simulink library "lib_Fin_Deflections"  (R2018b)
settings: Solver=VariableStepAuto  StartTime=0.0  StopTime=10.0  RelTol=1e-3
undefined symbols (not defined in the file or in its folder): FCC_PIX_Data, HIL_Data
settings Model: Creator=m.hiepp  LastModifiedBy=m.hiepp

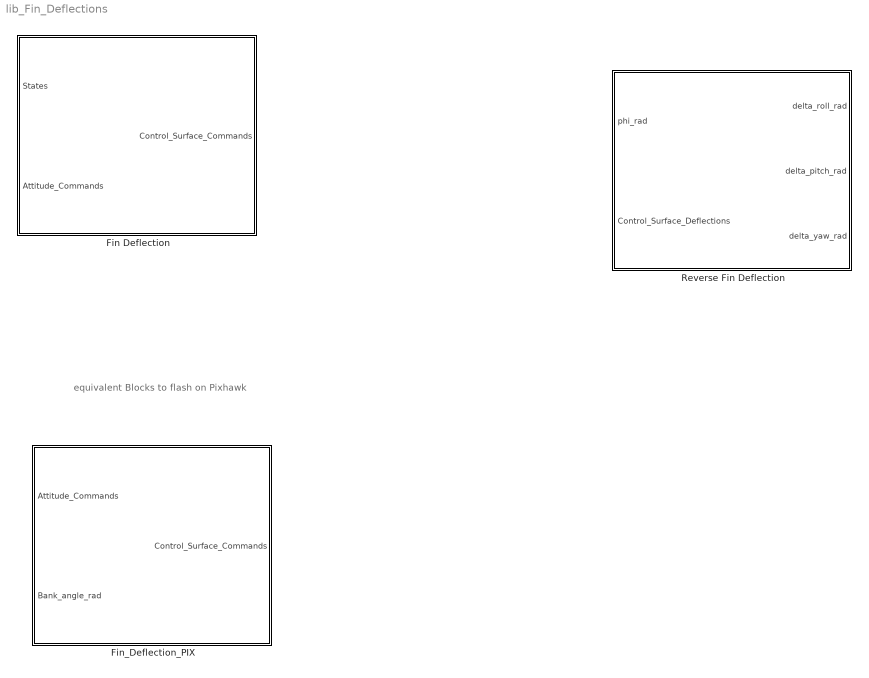
== system lib_Fin_Deflections ==
  note: equivalent Blocks to flash on Pixhawk
  Fin Deflection : Subsystem  mask{Control_Surfaces=HIL_Data.Control_Surfaces}
  Fin_Deflection_PIX : Subsystem
  Reverse Fin Deflection : Subsystem  mask{Control_Surfaces=HIL_Data.Control_Surfaces}

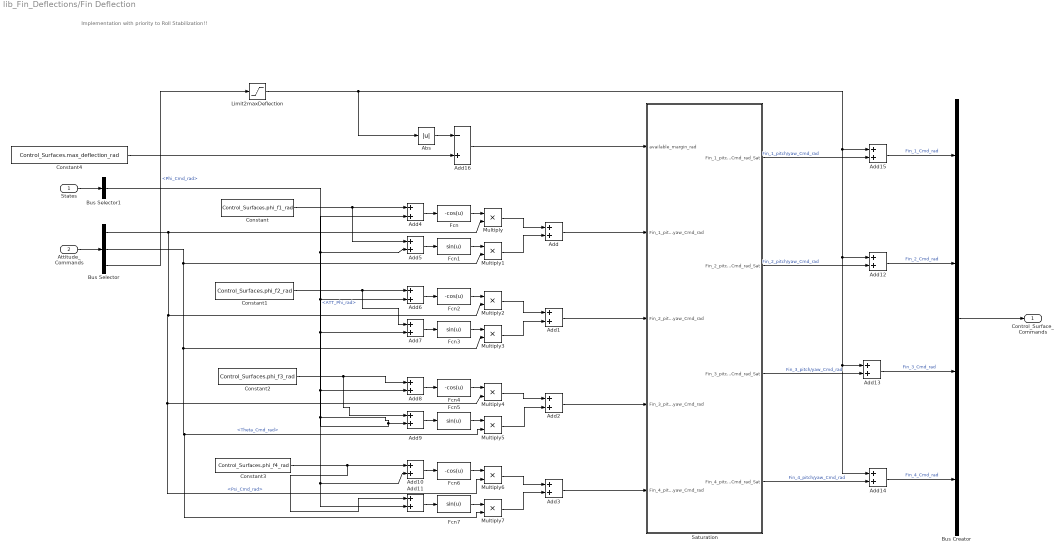
== system lib_Fin_Deflections/Fin Deflection ==
  note: Implementation with priority to Roll Stabilization!!
  States : Inport  OutDataTypeStr=Bus: States_Bus
  Attitude_Commands : Inport  Port=2  OutDataTypeStr=Bus: ATT_Cmd_Bus
  Abs : Abs
  Add{,1..15} (16 alike) : Sum
  Add16 : Sum  Inputs=-+
  Bus Creator : BusCreator  Inputs=4  OutDataTypeStr=Bus: Control_Surface_Cmd_Bus
  Bus Selector : BusSelector  OutputSignals=Psi_Cmd_rad,Theta_Cmd_rad,Phi_Cmd_rad
  Bus Selector1 : BusSelector  OutputSignals=Rigid_Body_States_Bus.Attitude_States_Bus.ATT_Euler_Bus.ATT_Phi_rad
  Constant : Constant  Value=Control_Surfaces.phi_f1_rad
  Constant1 : Constant  Value=Control_Surfaces.phi_f2_rad
  Constant2 : Constant  Value=Control_Surfaces.phi_f3_rad
  Constant3 : Constant  Value=Control_Surfaces.phi_f4_rad
  Constant4 : Constant  Value=Control_Surfaces.max_deflection_rad
  Fcn{,2,4,6} (4 alike) : Fcn  Expr=-cos(u)
  Fcn{1,3,5,7} (4 alike) : Fcn  Expr=sin(u)
  Limit2maxDeflection : Saturate  UpperLimit=Control_Surfaces.max_deflection_rad  LowerLimit=-Control_Surfaces.max_deflection_rad
  Multiply{,1..7} (8 alike) : Product
  Saturation : Subsystem
  Control_Surface_Commands : Outport  OutDataTypeStr=Bus: Control_Surface_Cmd_Bus
  wires:
  Add4/1 -> Fcn/1
  Fcn/1 -> Multiply/1
  Add5/1 -> Fcn1/1
  Fcn1/1 -> Multiply1/1
  Add7/1 -> Fcn3/1
  Add6/1 -> Fcn2/1
  Fcn2/1 -> Multiply2/1
  Fcn3/1 -> Multiply3/1
  Fcn5/1 -> Multiply5/1
  Add8/1 -> Fcn4/1
  Fcn4/1 -> Multiply4/1
  Add9/1 -> Fcn5/1
  Add11/1 -> Fcn7/1
  Fcn6/1 -> Multiply6/1
  Add10/1 -> Fcn6/1
  Fcn7/1 -> Multiply7/1
  Bus Selector/2 -> Multiply5/2, Multiply7/2, Multiply3/2, Multiply1/2  "<Theta_Cmd_rad>"
  Bus Selector/1 -> Multiply/2, Multiply6/2, Multiply4/2, Multiply2/2  "<Psi_Cmd_rad>"
  Multiply/1 -> Add/1
  Multiply1/1 -> Add/2
  Multiply2/1 -> Add1/1
  Multiply3/1 -> Add1/2
  Multiply4/1 -> Add2/1
  Multiply5/1 -> Add2/2
  Multiply6/1 -> Add3/1
  Multiply7/1 -> Add3/2
  Bus Selector1/1 -> Add11/2, Add10/2, Add7/2, Add4/2, Add5/2, Add6/2, Add8/2, Add9/2  "<ATT_Phi_rad>"
  Constant3/1 -> Add11/1, Add10/1
  Constant2/1 -> Add9/1, Add8/1
  Constant1/1 -> Add7/1, Add6/1
  Constant/1 -> Add5/1, Add4/1
  Attitude_Commands/1 -> Bus Selector/1
  Bus Creator/1 -> Control_Surface_Commands/1
  States/1 -> Bus Selector1/1
  Add/1 -> Saturation/2(Fin_1_pitch/yaw_Cmd_rad)
  Add1/1 -> Saturation/3(Fin_2_pitch/yaw_Cmd_rad)
  Add2/1 -> Saturation/4(Fin_3_pitch/yaw_Cmd_rad)
  Add3/1 -> Saturation/5(Fin_4_pitch/yaw_Cmd_rad)
  Add15/1 -> Bus Creator/1  "Fin_1_Cmd_rad"
  Add12/1 -> Bus Creator/2  "Fin_2_Cmd_rad"
  Add13/1 -> Bus Creator/3  "Fin_3_Cmd_rad"
  Add14/1 -> Bus Creator/4  "Fin_4_Cmd_rad"
  Bus Selector/3 -> Limit2maxDeflection/1  "<Phi_Cmd_rad>"
  Abs/1 -> Add16/1
  Constant4/1 -> Add16/2
  Add16/1 -> Saturation/1(available_margin_rad)
  Saturation/1(Fin_1_pitch/yaw_Cmd_rad_Sat) -> Add15/2  "Fin_1_pitch/yaw_Cmd_rad"
  Saturation/2(Fin_2_pitch/yaw_Cmd_rad_Sat) -> Add12/2  "Fin_2_pitch/yaw_Cmd_rad"
  Saturation/3(Fin_3_pitch/yaw_Cmd_rad_Sat) -> Add13/2  "Fin_3_pitch/yaw_Cmd_rad"
  Saturation/4(Fin_4_pitch/yaw_Cmd_rad_Sat) -> Add14/2  "Fin_4_pitch/yaw_Cmd_rad"
  Limit2maxDeflection/1 -> Abs/1, Add14/1, Add13/1, Add12/1, Add15/1

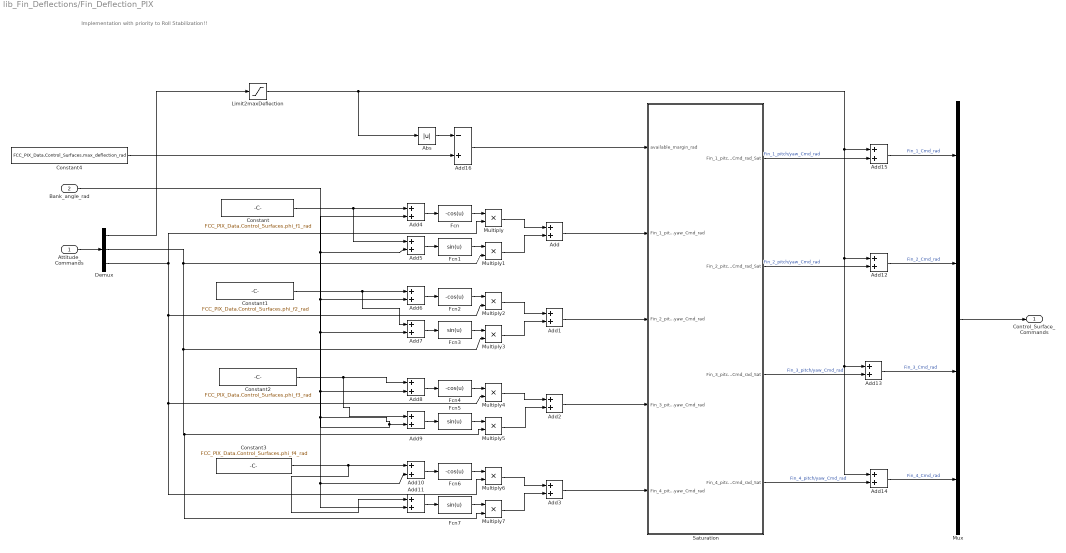
== system lib_Fin_Deflections/Fin_Deflection_PIX ==
  note: Implementation with priority to Roll Stabilization!!
  Attitude_Commands : Inport
  Bank_angle_rad : Inport  Port=2
  Abs : Abs
  Add{,1..15} (16 alike) : Sum
  Add16 : Sum  Inputs=-+
  Constant : Constant  Value=FCC_PIX_Data.Control_Surfaces.phi_f1_rad
  Constant1 : Constant  Value=FCC_PIX_Data.Control_Surfaces.phi_f2_rad
  Constant2 : Constant  Value=FCC_PIX_Data.Control_Surfaces.phi_f3_rad
  Constant3 : Constant  Value=FCC_PIX_Data.Control_Surfaces.phi_f4_rad
  Constant4 : Constant  Value=FCC_PIX_Data.Control_Surfaces.max_deflection_rad
  Demux : Demux  Outputs=3
  Fcn{,2,4,6} (4 alike) : Fcn  Expr=-cos(u)
  Fcn{1,3,5,7} (4 alike) : Fcn  Expr=sin(u)
  Limit2maxDeflection : Saturate  UpperLimit=FCC_PIX_Data.Control_Surfaces.max_deflection_rad  LowerLimit=-FCC_PIX_Data.Control_Surfaces.max_deflection_rad
  Multiply{,1..7} (8 alike) : Product
  Mux : Mux
  Saturation : Subsystem
  Control_Surface_Commands : Outport
  wires:
  Add4/1 -> Fcn/1
  Fcn/1 -> Multiply/1
  Add5/1 -> Fcn1/1
  Fcn1/1 -> Multiply1/1
  Add7/1 -> Fcn3/1
  Add6/1 -> Fcn2/1
  Fcn2/1 -> Multiply2/1
  Fcn3/1 -> Multiply3/1
  Fcn5/1 -> Multiply5/1
  Add8/1 -> Fcn4/1
  Fcn4/1 -> Multiply4/1
  Add9/1 -> Fcn5/1
  Add11/1 -> Fcn7/1
  Fcn6/1 -> Multiply6/1
  Add10/1 -> Fcn6/1
  Fcn7/1 -> Multiply7/1
  Demux/2 -> Multiply5/2, Multiply7/2, Multiply3/2, Multiply1/2
  Demux/3 -> Multiply/2, Multiply6/2, Multiply4/2, Multiply2/2
  Multiply/1 -> Add/1
  Multiply1/1 -> Add/2
  Multiply2/1 -> Add1/1
  Multiply3/1 -> Add1/2
  Multiply4/1 -> Add2/1
  Multiply5/1 -> Add2/2
  Multiply6/1 -> Add3/1
  Multiply7/1 -> Add3/2
  Bank_angle_rad/1 -> Add11/2, Add10/2, Add7/2, Add4/2, Add5/2, Add6/2, Add8/2, Add9/2
  Constant3/1 -> Add11/1, Add10/1
  Constant2/1 -> Add9/1, Add8/1
  Constant1/1 -> Add7/1, Add6/1
  Constant/1 -> Add5/1, Add4/1
  Attitude_Commands/1 -> Demux/1
  Mux/1 -> Control_Surface_Commands/1
  Add/1 -> Saturation/2(Fin_1_pitch/yaw_Cmd_rad)
  Add1/1 -> Saturation/3(Fin_2_pitch/yaw_Cmd_rad)
  Add2/1 -> Saturation/4(Fin_3_pitch/yaw_Cmd_rad)
  Add3/1 -> Saturation/5(Fin_4_pitch/yaw_Cmd_rad)
  Add15/1 -> Mux/1  "Fin_1_Cmd_rad"
  Add12/1 -> Mux/2  "Fin_2_Cmd_rad"
  Add13/1 -> Mux/3  "Fin_3_Cmd_rad"
  Add14/1 -> Mux/4  "Fin_4_Cmd_rad"
  Demux/1 -> Limit2maxDeflection/1
  Abs/1 -> Add16/1
  Constant4/1 -> Add16/2
  Add16/1 -> Saturation/1(available_margin_rad)
  Saturation/1(Fin_1_pitch/yaw_Cmd_rad_Sat) -> Add15/2  "Fin_1_pitch/yaw_Cmd_rad"
  Saturation/2(Fin_2_pitch/yaw_Cmd_rad_Sat) -> Add12/2  "Fin_2_pitch/yaw_Cmd_rad"
  Saturation/3(Fin_3_pitch/yaw_Cmd_rad_Sat) -> Add13/2  "Fin_3_pitch/yaw_Cmd_rad"
  Saturation/4(Fin_4_pitch/yaw_Cmd_rad_Sat) -> Add14/2  "Fin_4_pitch/yaw_Cmd_rad"
  Limit2maxDeflection/1 -> Abs/1, Add14/1, Add13/1, Add12/1, Add15/1

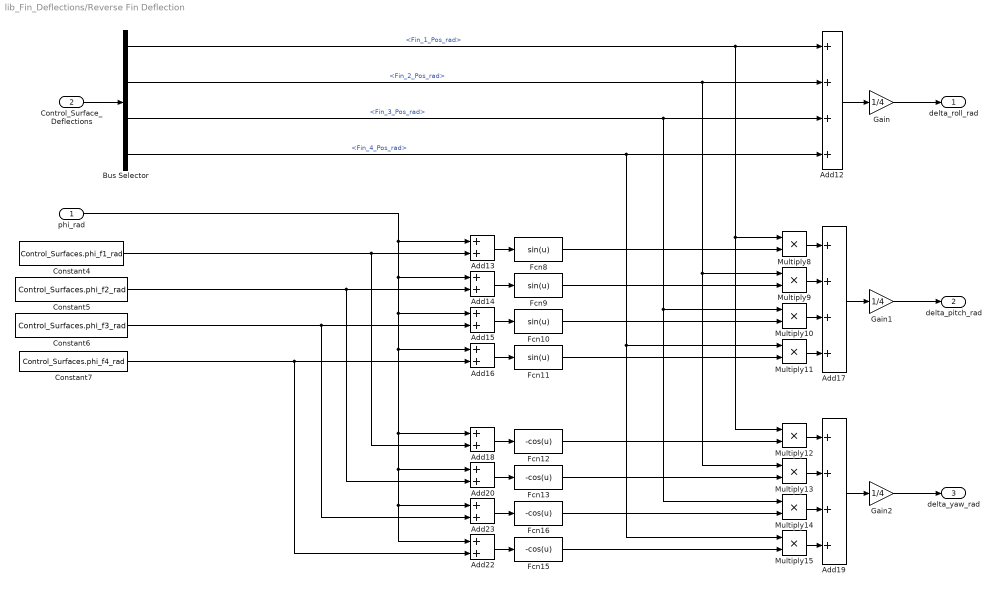
== system lib_Fin_Deflections/Reverse Fin Deflection ==
  phi_rad : Inport
  Control_Surface_Deflections : Inport  Port=2  OutDataTypeStr=Bus: Control_Surface_Deflections_Bus
  Add12 : Sum  Inputs=++++
  Add{13..16,18,20,22..23} (8 alike) : Sum
  Add17 : Sum  Inputs=++++
  Add19 : Sum  Inputs=++++
  Bus Selector : BusSelector  OutputSignals=Fin_1_Pos_rad,Fin_2_Pos_rad,Fin_3_Pos_rad,Fin_4_Pos_rad
  Constant4 : Constant  Value=Control_Surfaces.phi_f1_rad
  Constant5 : Constant  Value=Control_Surfaces.phi_f2_rad
  Constant6 : Constant  Value=Control_Surfaces.phi_f3_rad
  Constant7 : Constant  Value=Control_Surfaces.phi_f4_rad
  Fcn{8..11} (4 alike) : Fcn  Expr=sin(u)
  Fcn{12..13,15..16} (4 alike) : Fcn  Expr=-cos(u)
  Gain : Gain  Gain=1/4
  Gain1 : Gain  Gain=1/4
  Gain2 : Gain  Gain=1/4
  Multiply{8..15} (8 alike) : Product
  delta_roll_rad : Outport
  delta_pitch_rad : Outport  Port=2
  delta_yaw_rad : Outport  Port=3
  wires:
  Control_Surface_Deflections/1 -> Bus Selector/1
  Add12/1 -> Gain/1
  Gain/1 -> delta_roll_rad/1
  Bus Selector/1 -> Multiply12/1, Multiply8/1, Add12/1  "<Fin_1_Pos_rad>"
  Bus Selector/2 -> Multiply13/1, Multiply9/1, Add12/2  "<Fin_2_Pos_rad>"
  Bus Selector/3 -> Multiply10/1, Multiply14/1, Add12/3  "<Fin_3_Pos_rad>"
  Bus Selector/4 -> Multiply15/1, Multiply11/1, Add12/4  "<Fin_4_Pos_rad>"
  Add13/1 -> Fcn8/1
  Add14/1 -> Fcn9/1
  Add15/1 -> Fcn10/1
  Add16/1 -> Fcn11/1
  Add17/1 -> Gain1/1
  Gain1/1 -> delta_pitch_rad/1
  Add18/1 -> Fcn12/1
  Add19/1 -> Gain2/1
  Gain2/1 -> delta_yaw_rad/1
  Add20/1 -> Fcn13/1
  Add22/1 -> Fcn15/1
  Add23/1 -> Fcn16/1
  Multiply8/1 -> Add17/1
  Multiply15/1 -> Add19/4
  Multiply14/1 -> Add19/3
  Multiply13/1 -> Add19/2
  Multiply12/1 -> Add19/1
  Multiply11/1 -> Add17/4
  Multiply10/1 -> Add17/3
  Multiply9/1 -> Add17/2
  Fcn11/1 -> Multiply11/2
  Fcn10/1 -> Multiply10/2
  Fcn9/1 -> Multiply9/2
  Fcn8/1 -> Multiply8/2
  Fcn15/1 -> Multiply15/2
  Fcn16/1 -> Multiply14/2
  Fcn13/1 -> Multiply13/2
  Fcn12/1 -> Multiply12/2
  Constant4/1 -> Add18/2, Add13/2
  Constant5/1 -> Add20/2, Add14/2
  Constant6/1 -> Add23/2, Add15/2
  Constant7/1 -> Add22/2, Add16/2
  phi_rad/1 -> Add15/1, Add16/1, Add23/1, Add22/1, Add20/1, Add18/1, Add14/1, Add13/1

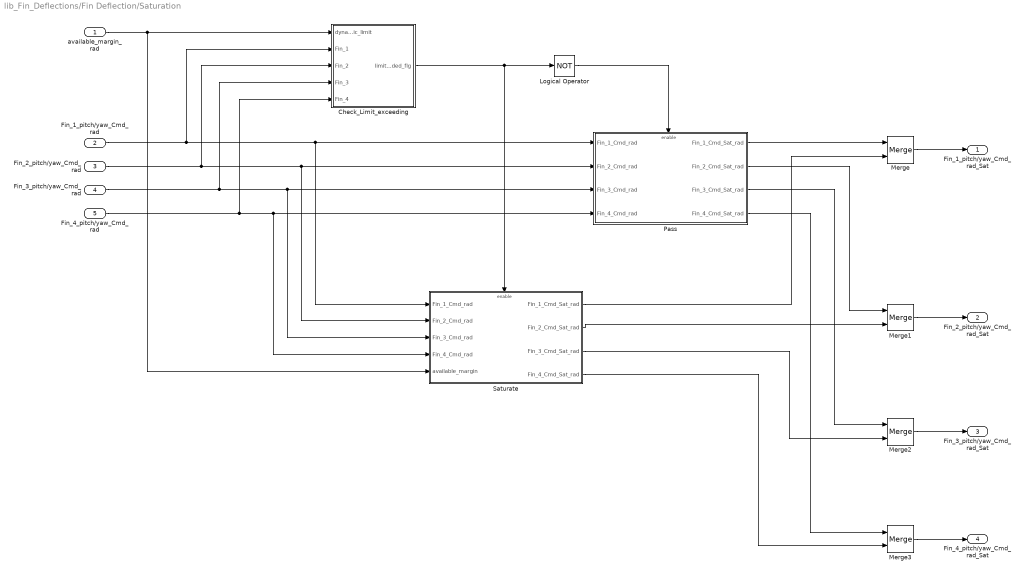
== system lib_Fin_Deflections/Fin Deflection/Saturation ==
  available_margin_rad : Inport
  Fin_1_pitch/yaw_Cmd_rad : Inport  Port=2
  Fin_2_pitch/yaw_Cmd_rad : Inport  Port=3
  Fin_3_pitch/yaw_Cmd_rad : Inport  Port=4
  Fin_4_pitch/yaw_Cmd_rad : Inport  Port=5
  Check_Limit_exceeding : Subsystem
  Logical Operator : Logic  Operator=NOT  AllPortsSameDT=off  OutDataTypeStr=boolean
  Merge{,1..3} (4 alike) : Merge
  Pass : Subsystem
  Saturate : Subsystem
  Fin_1_pitch/yaw_Cmd_rad_Sat : Outport
  Fin_2_pitch/yaw_Cmd_rad_Sat : Outport  Port=2
  Fin_3_pitch/yaw_Cmd_rad_Sat : Outport  Port=3
  Fin_4_pitch/yaw_Cmd_rad_Sat : Outport  Port=4
  wires:
  Fin_1_pitch/yaw_Cmd_rad/1 -> Check_Limit_exceeding/2(Fin_1), Saturate/1(Fin_1_Cmd_rad), Pass/1(Fin_1_Cmd_rad)
  Fin_2_pitch/yaw_Cmd_rad/1 -> Check_Limit_exceeding/3(Fin_2), Pass/2(Fin_2_Cmd_rad), Saturate/2(Fin_2_Cmd_rad)
  Fin_3_pitch/yaw_Cmd_rad/1 -> Check_Limit_exceeding/4(Fin_3), Pass/3(Fin_3_Cmd_rad), Saturate/3(Fin_3_Cmd_rad)
  Fin_4_pitch/yaw_Cmd_rad/1 -> Check_Limit_exceeding/5(Fin_4), Saturate/4(Fin_4_Cmd_rad), Pass/4(Fin_4_Cmd_rad)
  Merge/1 -> Fin_1_pitch/yaw_Cmd_rad_Sat/1
  Merge3/1 -> Fin_4_pitch/yaw_Cmd_rad_Sat/1
  Merge1/1 -> Fin_2_pitch/yaw_Cmd_rad_Sat/1
  Check_Limit_exceeding/1(limit_exceeded_flg) -> Saturate/Enable, Logical Operator/1
  Logical Operator/1 -> Pass/Enable
  Merge2/1 -> Fin_3_pitch/yaw_Cmd_rad_Sat/1
  Pass/1(Fin_1_Cmd_Sat_rad) -> Merge/1
  Pass/2(Fin_2_Cmd_Sat_rad) -> Merge1/1
  Pass/3(Fin_3_Cmd_Sat_rad) -> Merge2/1
  Pass/4(Fin_4_Cmd_Sat_rad) -> Merge3/1
  Saturate/1(Fin_1_Cmd_Sat_rad) -> Merge/2
  Saturate/2(Fin_2_Cmd_Sat_rad) -> Merge1/2
  Saturate/3(Fin_3_Cmd_Sat_rad) -> Merge2/2
  Saturate/4(Fin_4_Cmd_Sat_rad) -> Merge3/2
  available_margin_rad/1 -> Saturate/5(available_margin), Check_Limit_exceeding/1(dynamic_limit)

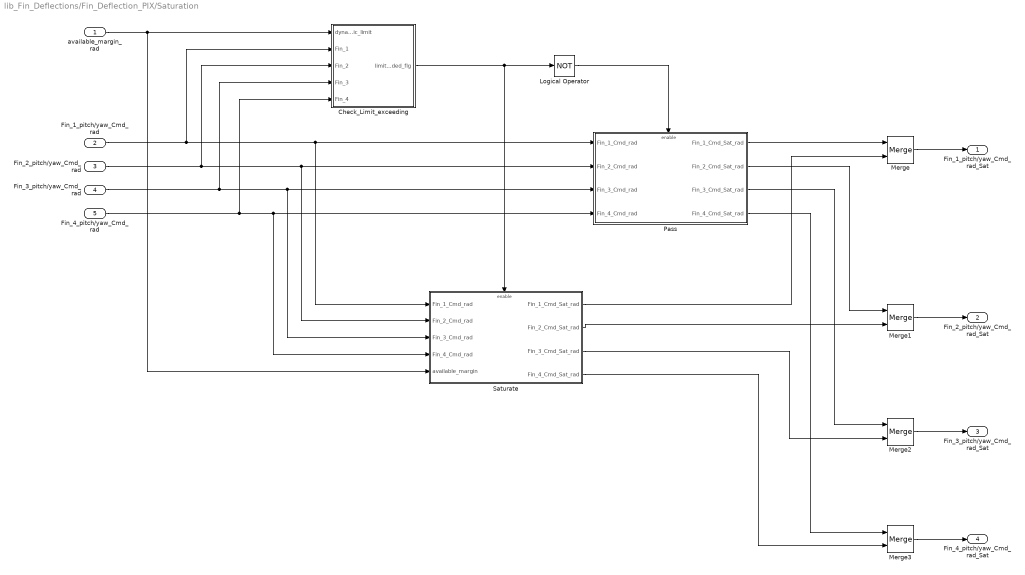
== system lib_Fin_Deflections/Fin_Deflection_PIX/Saturation ==
  available_margin_rad : Inport
  Fin_1_pitch/yaw_Cmd_rad : Inport  Port=2
  Fin_2_pitch/yaw_Cmd_rad : Inport  Port=3
  Fin_3_pitch/yaw_Cmd_rad : Inport  Port=4
  Fin_4_pitch/yaw_Cmd_rad : Inport  Port=5
  Check_Limit_exceeding : Subsystem
  Logical Operator : Logic  Operator=NOT  AllPortsSameDT=off  OutDataTypeStr=boolean
  Merge{,1..3} (4 alike) : Merge
  Pass : Subsystem
  Saturate : Subsystem
  Fin_1_pitch/yaw_Cmd_rad_Sat : Outport
  Fin_2_pitch/yaw_Cmd_rad_Sat : Outport  Port=2
  Fin_3_pitch/yaw_Cmd_rad_Sat : Outport  Port=3
  Fin_4_pitch/yaw_Cmd_rad_Sat : Outport  Port=4
  wires:
  Fin_1_pitch/yaw_Cmd_rad/1 -> Check_Limit_exceeding/2(Fin_1), Saturate/1(Fin_1_Cmd_rad), Pass/1(Fin_1_Cmd_rad)
  Fin_2_pitch/yaw_Cmd_rad/1 -> Check_Limit_exceeding/3(Fin_2), Pass/2(Fin_2_Cmd_rad), Saturate/2(Fin_2_Cmd_rad)
  Fin_3_pitch/yaw_Cmd_rad/1 -> Check_Limit_exceeding/4(Fin_3), Pass/3(Fin_3_Cmd_rad), Saturate/3(Fin_3_Cmd_rad)
  Fin_4_pitch/yaw_Cmd_rad/1 -> Check_Limit_exceeding/5(Fin_4), Saturate/4(Fin_4_Cmd_rad), Pass/4(Fin_4_Cmd_rad)
  Merge/1 -> Fin_1_pitch/yaw_Cmd_rad_Sat/1
  Merge3/1 -> Fin_4_pitch/yaw_Cmd_rad_Sat/1
  Merge1/1 -> Fin_2_pitch/yaw_Cmd_rad_Sat/1
  Check_Limit_exceeding/1(limit_exceeded_flg) -> Saturate/Enable, Logical Operator/1
  Logical Operator/1 -> Pass/Enable
  Merge2/1 -> Fin_3_pitch/yaw_Cmd_rad_Sat/1
  Pass/1(Fin_1_Cmd_Sat_rad) -> Merge/1
  Pass/2(Fin_2_Cmd_Sat_rad) -> Merge1/1
  Pass/3(Fin_3_Cmd_Sat_rad) -> Merge2/1
  Pass/4(Fin_4_Cmd_Sat_rad) -> Merge3/1
  Saturate/1(Fin_1_Cmd_Sat_rad) -> Merge/2
  Saturate/2(Fin_2_Cmd_Sat_rad) -> Merge1/2
  Saturate/3(Fin_3_Cmd_Sat_rad) -> Merge2/2
  Saturate/4(Fin_4_Cmd_Sat_rad) -> Merge3/2
  available_margin_rad/1 -> Saturate/5(available_margin), Check_Limit_exceeding/1(dynamic_limit)

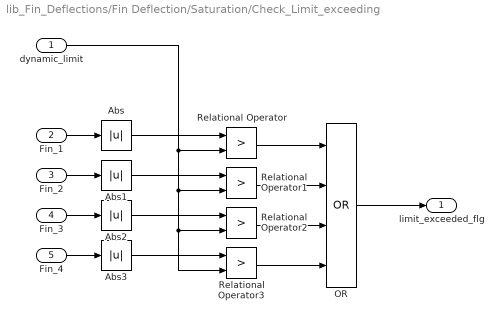
== system lib_Fin_Deflections/Fin Deflection/Saturation/Check_Limit_exceeding ==
  dynamic_limit : Inport
  Fin_1 : Inport  Port=2
  Fin_2 : Inport  Port=3
  Fin_3 : Inport  Port=4
  Fin_4 : Inport  Port=5
  Abs{,1..3} (4 alike) : Abs  ZeroCross=off
  OR : Logic  Operator=OR  Inputs=4  IconShape=distinctive  AllPortsSameDT=off  OutDataTypeStr=boolean
  Relational Operator{,1..3} (4 alike) : RelationalOperator  Operator=>  OutDataTypeStr=boolean  RndMeth=Simplest
  limit_exceeded_flg : Outport
  wires:
  OR/1 -> limit_exceeded_flg/1
  Fin_4/1 -> Abs3/1
  Fin_3/1 -> Abs2/1
  Fin_2/1 -> Abs1/1
  Fin_1/1 -> Abs/1
  Relational Operator/1 -> OR/1
  Relational Operator1/1 -> OR/2
  Relational Operator2/1 -> OR/3
  Relational Operator3/1 -> OR/4
  Abs/1 -> Relational Operator/1
  Abs1/1 -> Relational Operator1/1
  Abs2/1 -> Relational Operator2/1
  Abs3/1 -> Relational Operator3/1
  dynamic_limit/1 -> Relational Operator/2, Relational Operator3/2, Relational Operator2/2, Relational Operator1/2

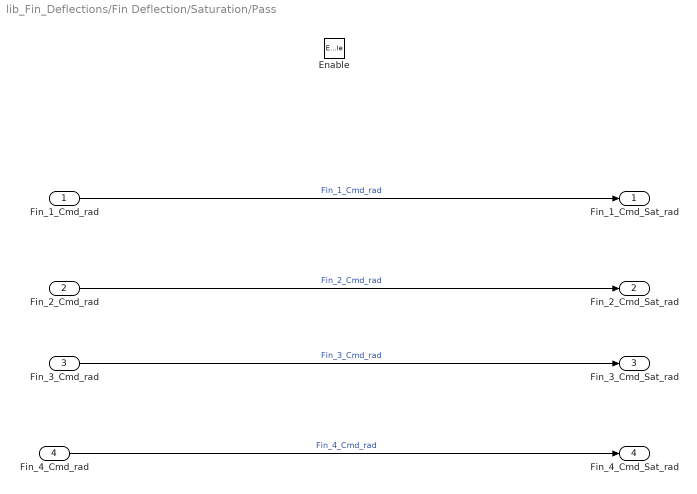
== system lib_Fin_Deflections/Fin Deflection/Saturation/Pass ==
  Fin_1_Cmd_rad : Inport
  Fin_2_Cmd_rad : Inport  Port=2
  Fin_3_Cmd_rad : Inport  Port=3
  Fin_4_Cmd_rad : Inport  Port=4
  Enable : EnablePort
  Fin_1_Cmd_Sat_rad : Outport
  Fin_2_Cmd_Sat_rad : Outport  Port=2
  Fin_3_Cmd_Sat_rad : Outport  Port=3
  Fin_4_Cmd_Sat_rad : Outport  Port=4
  wires:
  Fin_2_Cmd_rad/1 -> Fin_2_Cmd_Sat_rad/1  "Fin_2_Cmd_rad"
  Fin_1_Cmd_rad/1 -> Fin_1_Cmd_Sat_rad/1  "Fin_1_Cmd_rad"
  Fin_4_Cmd_rad/1 -> Fin_4_Cmd_Sat_rad/1  "Fin_4_Cmd_rad"
  Fin_3_Cmd_rad/1 -> Fin_3_Cmd_Sat_rad/1  "Fin_3_Cmd_rad"

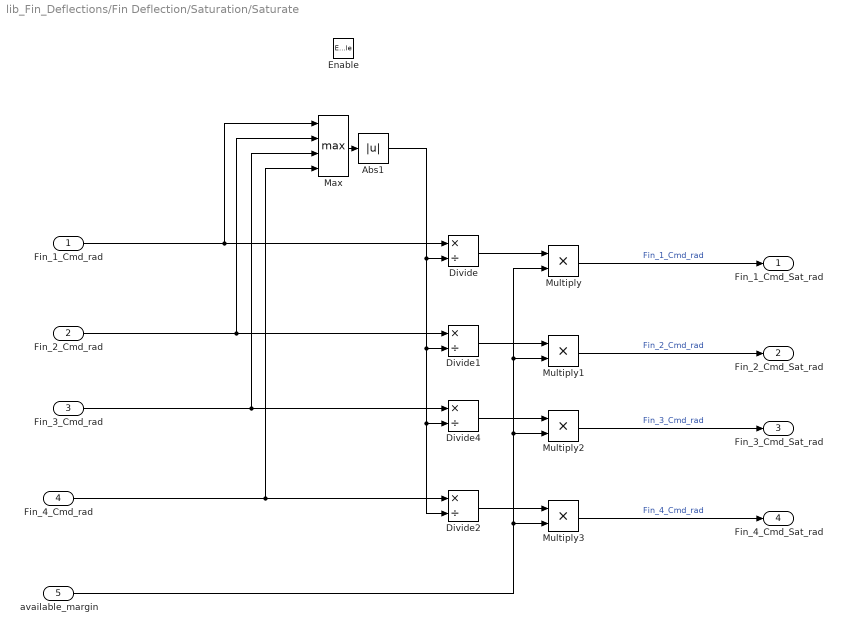
== system lib_Fin_Deflections/Fin Deflection/Saturation/Saturate ==
  Fin_1_Cmd_rad : Inport
  Fin_2_Cmd_rad : Inport  Port=2
  Fin_3_Cmd_rad : Inport  Port=3
  Fin_4_Cmd_rad : Inport  Port=4
  available_margin : Inport  Port=5
  Enable : EnablePort
  Abs1 : Abs
  Divide{,1..2,4} (4 alike) : Product  Inputs=*/
  Max : MinMax  Function=max  Inputs=4
  Multiply{,1..3} (4 alike) : Product
  Fin_1_Cmd_Sat_rad : Outport
  Fin_2_Cmd_Sat_rad : Outport  Port=2
  Fin_3_Cmd_Sat_rad : Outport  Port=3
  Fin_4_Cmd_Sat_rad : Outport  Port=4
  wires:
  Fin_1_Cmd_rad/1 -> Max/1, Divide/1
  Divide/1 -> Multiply/1
  Divide1/1 -> Multiply1/1
  Divide2/1 -> Multiply3/1
  Abs1/1 -> Divide2/2, Divide4/2, Divide1/2, Divide/2
  Multiply1/1 -> Fin_2_Cmd_Sat_rad/1  "Fin_2_Cmd_rad"
  Fin_2_Cmd_rad/1 -> Max/2, Divide1/1
  Fin_4_Cmd_rad/1 -> Max/4, Divide2/1
  Fin_3_Cmd_rad/1 -> Max/3, Divide4/1
  Max/1 -> Abs1/1
  Divide4/1 -> Multiply2/1
  Multiply/1 -> Fin_1_Cmd_Sat_rad/1  "Fin_1_Cmd_rad"
  Multiply3/1 -> Fin_4_Cmd_Sat_rad/1  "Fin_4_Cmd_rad"
  Multiply2/1 -> Fin_3_Cmd_Sat_rad/1  "Fin_3_Cmd_rad"
  available_margin/1 -> Multiply/2, Multiply1/2, Multiply2/2, Multiply3/2

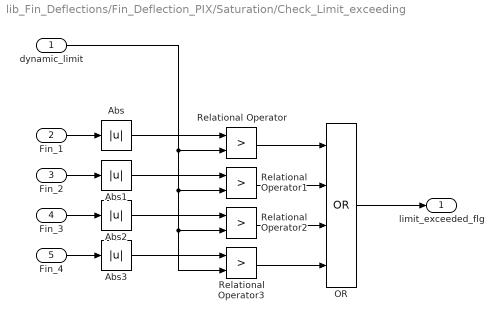
== system lib_Fin_Deflections/Fin_Deflection_PIX/Saturation/Check_Limit_exceeding ==
  dynamic_limit : Inport
  Fin_1 : Inport  Port=2
  Fin_2 : Inport  Port=3
  Fin_3 : Inport  Port=4
  Fin_4 : Inport  Port=5
  Abs{,1..3} (4 alike) : Abs
  OR : Logic  Operator=OR  Inputs=4  IconShape=distinctive  AllPortsSameDT=off  OutDataTypeStr=boolean
  Relational Operator{,1..3} (4 alike) : RelationalOperator  Operator=>  OutDataTypeStr=boolean  RndMeth=Simplest
  limit_exceeded_flg : Outport
  wires:
  OR/1 -> limit_exceeded_flg/1
  Fin_4/1 -> Abs3/1
  Fin_3/1 -> Abs2/1
  Fin_2/1 -> Abs1/1
  Fin_1/1 -> Abs/1
  Relational Operator/1 -> OR/1
  Relational Operator1/1 -> OR/2
  Relational Operator2/1 -> OR/3
  Relational Operator3/1 -> OR/4
  Abs/1 -> Relational Operator/1
  Abs1/1 -> Relational Operator1/1
  Abs2/1 -> Relational Operator2/1
  Abs3/1 -> Relational Operator3/1
  dynamic_limit/1 -> Relational Operator/2, Relational Operator3/2, Relational Operator2/2, Relational Operator1/2

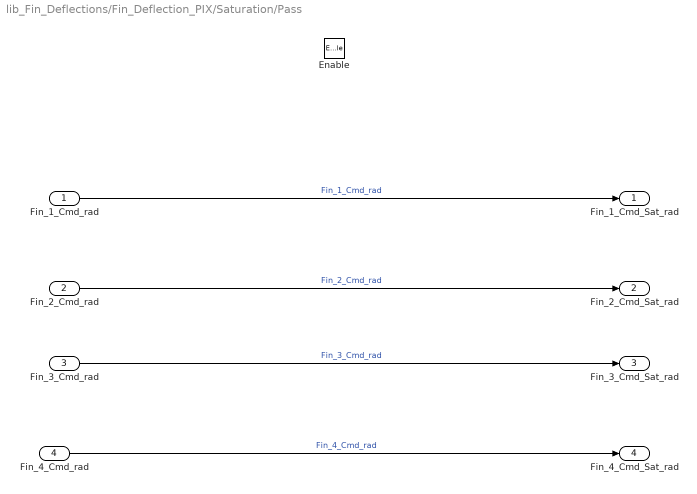
== system lib_Fin_Deflections/Fin_Deflection_PIX/Saturation/Pass ==
  Fin_1_Cmd_rad : Inport
  Fin_2_Cmd_rad : Inport  Port=2
  Fin_3_Cmd_rad : Inport  Port=3
  Fin_4_Cmd_rad : Inport  Port=4
  Enable : EnablePort
  Fin_1_Cmd_Sat_rad : Outport
  Fin_2_Cmd_Sat_rad : Outport  Port=2
  Fin_3_Cmd_Sat_rad : Outport  Port=3
  Fin_4_Cmd_Sat_rad : Outport  Port=4
  wires:
  Fin_2_Cmd_rad/1 -> Fin_2_Cmd_Sat_rad/1  "Fin_2_Cmd_rad"
  Fin_1_Cmd_rad/1 -> Fin_1_Cmd_Sat_rad/1  "Fin_1_Cmd_rad"
  Fin_4_Cmd_rad/1 -> Fin_4_Cmd_Sat_rad/1  "Fin_4_Cmd_rad"
  Fin_3_Cmd_rad/1 -> Fin_3_Cmd_Sat_rad/1  "Fin_3_Cmd_rad"

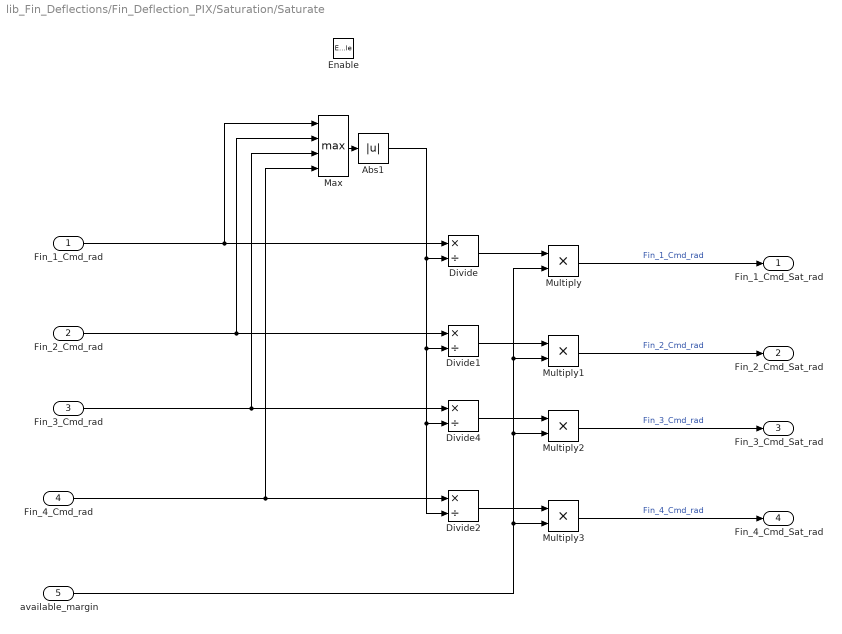
== system lib_Fin_Deflections/Fin_Deflection_PIX/Saturation/Saturate ==
  Fin_1_Cmd_rad : Inport
  Fin_2_Cmd_rad : Inport  Port=2
  Fin_3_Cmd_rad : Inport  Port=3
  Fin_4_Cmd_rad : Inport  Port=4
  available_margin : Inport  Port=5
  Enable : EnablePort
  Abs1 : Abs
  Divide{,1..2,4} (4 alike) : Product  Inputs=*/
  Max : MinMax  Function=max  Inputs=4
  Multiply{,1..3} (4 alike) : Product
  Fin_1_Cmd_Sat_rad : Outport
  Fin_2_Cmd_Sat_rad : Outport  Port=2
  Fin_3_Cmd_Sat_rad : Outport  Port=3
  Fin_4_Cmd_Sat_rad : Outport  Port=4
  wires:
  Fin_1_Cmd_rad/1 -> Max/1, Divide/1
  Divide/1 -> Multiply/1
  Divide1/1 -> Multiply1/1
  Divide2/1 -> Multiply3/1
  Abs1/1 -> Divide2/2, Divide4/2, Divide1/2, Divide/2
  Multiply1/1 -> Fin_2_Cmd_Sat_rad/1  "Fin_2_Cmd_rad"
  Fin_2_Cmd_rad/1 -> Max/2, Divide1/1
  Fin_4_Cmd_rad/1 -> Max/4, Divide2/1
  Fin_3_Cmd_rad/1 -> Max/3, Divide4/1
  Max/1 -> Abs1/1
  Divide4/1 -> Multiply2/1
  Multiply/1 -> Fin_1_Cmd_Sat_rad/1  "Fin_1_Cmd_rad"
  Multiply3/1 -> Fin_4_Cmd_Sat_rad/1  "Fin_4_Cmd_rad"
  Multiply2/1 -> Fin_3_Cmd_Sat_rad/1  "Fin_3_Cmd_rad"
  available_margin/1 -> Multiply/2, Multiply1/2, Multiply2/2, Multiply3/2
